simulink library "BLE_Library"  (R2017b)
settings: Solver=VariableStepAuto  StartTime=0.0  StopTime=10.0  RelTol=1e-3
values from neighbouring files (symbols this model uses):
  D = D/ScaleCoefficient    [BLE_PostLoad.m]    (also in new_BLE_model.m = zeros(N_BLE,N_BLE+1))
undefined symbols (not defined in the file or in its folder): ADV_IND_AccA, ADV_IND_id, BT_Hop_Separation, BT_Samples_Per_Symbol, CONNECT_IND_id, CONNECT_IND_length, F3B672D172DF, F506B10B1B3E, Header, LL_DATA_EMPTY_length, LL_DATA_id, magnitude, Payload, Preamble, Slot_Ts, T_IFS
libraries: BLE_Library x56, simulink x39, commutil2 x29, dspindex x17, commdigbbndfm2 x5, dspsigops x2, commrandsrc3 x2, dspstat3 x2, dspsrcs4 x1, dsparch4 x1, commdigbbndcpm2 x1
(part 3 of 5)

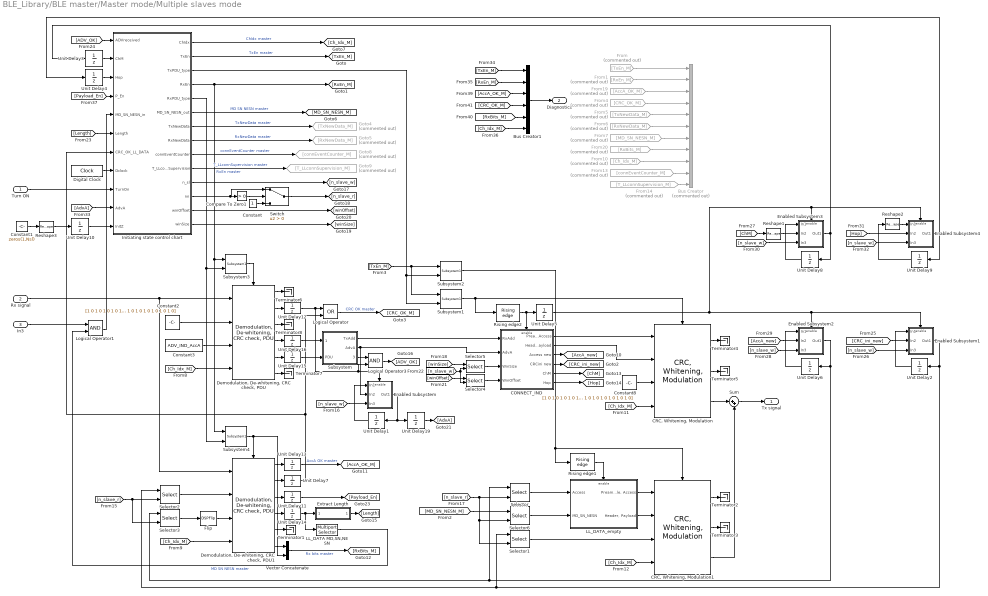
== system BLE_Library/BLE master/Master mode/Multiple slaves mode ==
  Turn ON : Inport
  Rx signal : Inport  Port=2
  In3 : Inport  Port=3
  Bus Creator : BusCreator  Commented=on  Inputs=11
  Bus Creator1 : BusCreator  Inputs=6
  CONNECT_IND : Subsystem
  "CRC, Whitening, Modulation" : BLE_Library/CRC, Whitening,  Modulation
  "CRC, Whitening, Modulation1" : BLE_Library/CRC, Whitening,  Modulation
  Compare To Zero1 : simulink/Logic and Bit Operations/Compare To Zero  relop=>  OutDataTypeStr=boolean
  Constant : Constant  SampleTime=-1
  Constant1 : Constant  Value=zeros(1,Nsl)  OutDataTypeStr=double  SampleTime=Slot_Ts
  Constant2 : Constant  Value=[1 0 1 0 1 0 1 0 1 0 1 0 1 0 1 0 1 0 1 0 1 0 1 0]  OutDataTypeStr=boolean  SampleTime=Slot_Ts
  Constant3 : Constant  Value=ADV_IND_AccA  VectorParams1D=off  SampleTime=Slot_Ts
  Constant8 : Constant  Value=[1 0 1 0 1 0 1 0 1 0 1 0 1 0 1 0 1 0 1 0 1 0 1 0]  OutDataTypeStr=boolean  SampleTime=Slot_Ts
  "Demodulation, De-whitening, CRC check, PDU" : BLE_Library/Demodulation, De-whitening, CRC check, PDU  PDU_Length=112 %ADV_DIRECT_IND: 2+6+6 octets (H,AdvA,TargetA)  N_after=136 %max PDU length + CRC
  "Demodulation, De-whitening, CRC check, PDU1" : BLE_Library/Demodulation, De-whitening, CRC check, PDU  PDU_Length=2 %PDU is not required  N_after=2080 %max PDU length + CRC: 16 + 255*8 + 24
  Digital Clock : DigitalClock  SampleTime=Slot_Ts
  Enabled Subsystem : Subsystem  TreatAsAtomicUnit=on
  Enabled Subsystem1 : Subsystem  TreatAsAtomicUnit=on
  Enabled Subsystem2 : Subsystem  TreatAsAtomicUnit=on
  Enabled Subsystem3 : Subsystem  TreatAsAtomicUnit=on
  Enabled Subsystem4 : Subsystem  TreatAsAtomicUnit=on
  Extract Length : Subsystem
      mask Display: disp('Extract length')
  Flip : DSPFlip
  From : From  Commented=on  GotoTag=TxEn_M
  From1 : From  Commented=on  GotoTag=RxEn_M
  From10 : From  Commented=on  GotoTag=Ch_Idx_M
  From13 : From  Commented=on  GotoTag=connEventCounter_M
  From14 : From  Commented=on  GotoTag=T_LLconnSupervision_M
  From19 : From  Commented=on  GotoTag=AccA_OK_M
  From20 : From  Commented=on  GotoTag=RxBits_M
  From4 : From  Commented=on  GotoTag=CRC_OK_M
  From5 : From  Commented=on  GotoTag=TxNewData_M
  From6 : From  Commented=on  GotoTag=RxNewData_M
  From7 : From  Commented=on  GotoTag=MD_SN_NESN_M
  Goto4 : Goto  Commented=on  GotoTag=TxNewData_M
  Goto5 : Goto  Commented=on  GotoTag=RxNewData_M
  Goto8 : Goto  Commented=on  GotoTag=connEventCounter_M
  Goto9 : Goto  Commented=on  GotoTag=T_LLconnSupervision_M
  Initiating state control chart : Stateflow chart  TreatAsAtomicUnit=on
  LL_DATA MD,SN,NESN : dspindex/Multiport Selector  rowsOrCols=Rows  idxCellArray={12:14}  idxErrMode=Clip Index
  LL_DATA_empty : Subsystem
  Logical Operator : Logic  Operator=OR  AllPortsSameDT=off  OutDataTypeStr=boolean
  Logical Operator1 : Logic  AllPortsSameDT=off  OutDataTypeStr=boolean
  Logical Operator3 : Logic  AllPortsSameDT=off  OutDataTypeStr=boolean
  Reshape1 : Reshape  OutputDimensionality=Column vector (2-D)
  Reshape2 : Reshape  OutputDimensionality=Row vector (2-D)
  Reshape3 : Reshape  OutputDimensionality=Row vector (2-D)
  Rising edge1 : BLE_Library/Rising edge  SystemSampleTime=-1
  Rising edge2 : BLE_Library/Rising edge  SystemSampleTime=-1
  Selector{,1..6} (7 alike) : Selector  NumberOfDimensions=2  InputPortWidth=3  IndexOptions=Select all,Index vector (port)  Indices=[1 3],2  OutputSizes=1,1
  Subsystem : Subsystem
  Subsystem1 : BLE_Library/Subsystem1  PDU_type=CONNECT_IND_id
  Subsystem2 : BLE_Library/Subsystem1  PDU_type=LL_DATA_id
  Subsystem3 : BLE_Library/Subsystem1  PDU_type=ADV_IND_id
  Subsystem4 : BLE_Library/Subsystem1  PDU_type=LL_DATA_id
  Sum : Sum  Inputs=|++
  Switch : Switch  Criteria=u2 > Threshold
  Terminator{1..8} (8 alike) : Terminator
  Unit Delay1 : UnitDelay  InitialCondition=zeros(48,Nsl)  SampleTime=Slot_Ts
  Unit Delay{3..5,7,10..16,19} (12 alike) : UnitDelay  SampleTime=Slot_Ts
  Unit Delay2 : UnitDelay  InitialCondition=zeros(24,Nsl)  SampleTime=Slot_Ts
  Unit Delay6 : UnitDelay  InitialCondition=zeros(32,Nsl)  SampleTime=Slot_Ts
  Unit Delay8 : UnitDelay  InitialCondition=zeros(40,Nsl)  SampleTime=Slot_Ts
  Unit Delay9 : UnitDelay  InitialCondition=zeros(1,Nsl)  SampleTime=Slot_Ts
  Vector Concatenate : Concatenate
  Tx signal : Outport
  Diagnostics : Outport  Port=2
  wires:
  "Demodulation, De-whitening, CRC check, PDU1"/2 -> Unit Delay7/1
  Subsystem4/1 -> "Demodulation, De-whitening, CRC check, PDU1"/Enable, Vector Concatenate/2
  Selector4/1 -> CONNECT_IND/4(WinOffset)
  [n_slave_w] -> Enabled Subsystem/3(In3)
  "CRC, Whitening, Modulation1"/2 -> Terminator3/1
  [Ch_Idx_M] -> "CRC, Whitening, Modulation1"/4
  Initiating state control chart/8(RxNewData) -> Goto5/1  "RxNewData master"
  Initiating state control chart/11(n_sl) -> [n_slave_w]
  "Demodulation, De-whitening, CRC check, PDU"/2 -> Unit Delay12/1
  Unit Delay12/1 -> Enabled Subsystem/Enable, Logical Operator3/2, Logical Operator/1
  Initiating state control chart/10(T_LLconnSupervision) -> Goto9/1  "T_LLconnSupervision master"
  Unit Delay19/1 -> [AdvA]
  [n_slave_w] -> Enabled Subsystem2/3(In3)
  Selector/1 -> LL_DATA_empty/1(Access)
  From/1 -> Bus Creator/1
  Subsystem/2(AdvA) -> CONNECT_IND/2(AdvA), Enabled Subsystem/2(In2)
  "Demodulation, De-whitening, CRC check, PDU"/1 -> Terminator6/1
  Initiating state control chart/9(connEventCounter) -> Goto8/1  "connEventCounter master"
  Sum/1 -> Tx signal/1
  CONNECT_IND/6(Hop) -> [Hop]
  [TxEn_M] -> Bus Creator1/1
  Enabled Subsystem/1(Out1) -> Unit Delay1/1, Unit Delay19/1
  Rising edge1/1 -> LL_DATA_empty/Enable
  Initiating state control chart/1(ChIdx) -> [Ch_Idx_M]  "ChIdx master"
  [RxBits_M] -> Bus Creator1/5
  Initiating state control chart/3(TxPDU_type) -> Subsystem2/2, Subsystem1/2
  LL_DATA_empty/1("Preamble, Access") -> "CRC, Whitening, Modulation1"/1
  Initiating state control chart/4(RxEn) -> [RxEn_M], Subsystem4/1, Subsystem3/1  "RxEn master"
  Subsystem/1(TxAdd) -> CONNECT_IND/1(RxAdd)
  Initiating state control chart/5(RxPDU_type) -> Subsystem4/2, Subsystem3/2
  From13/1 -> Bus Creator/10
  Initiating state control chart/6(MD_SN_NESN_out) -> [MD_SN_NESN_M]  "MD SN NESN master"
  [winOffset] -> Selector4/1
  From14/1 -> Bus Creator/11
  From4/1 -> Bus Creator/4
  Initiating state control chart/14(winSize) -> [winSize]
  [AccA_new] -> Enabled Subsystem2/2(In2)
  From20/1 -> Bus Creator/8
  Unit Delay6/1 -> Enabled Subsystem2/1(In1)
  "Demodulation, De-whitening, CRC check, PDU1"/1 -> Unit Delay13/1
  [Hop] -> Enabled Subsystem4/2(In2)
  Constant8/1 -> "CRC, Whitening, Modulation"/3
  Constant1/1 -> Reshape3/1
  Enabled Subsystem1/1(Out1) -> Unit Delay2/1, Selector2/1, Selector1/1
  Unit Delay7/1 -> Logical Operator/2, Initiating state control chart/7(CRC_OK_LL_DATA)
  Digital Clock/1 -> Initiating state control chart/8(Dclock)
  CONNECT_IND/4(CRCini new) -> [CRC_ini_new]
  Selector6/1 -> LL_DATA_empty/2(MD_SN_NESN)
  Initiating state control chart/13(winOffset) -> [winOffset]
  Enabled Subsystem3/1(Out1) -> Unit Delay3/1, Unit Delay8/1
  [n_slave_w] -> Enabled Subsystem4/3(In3)
  Unit Delay5/1 -> Enabled Subsystem2/Enable, Enabled Subsystem1/Enable, Enabled Subsystem4/Enable, Enabled Subsystem3/Enable
  Unit Delay16/1 -> Subsystem/1(Header)
  Compare To Zero1/1 -> Switch/2
  Enabled Subsystem4/1(Out1) -> Unit Delay4/1, Unit Delay9/1
  Enabled Subsystem2/1(Out1) -> Selector/1, Selector3/1, Unit Delay6/1
  [AccA_OK_M] -> Bus Creator1/3
  CONNECT_IND/5(ChM) -> [ChM]
  CONNECT_IND/3(Access new) -> [AccA_new]
  [MD_SN_NESN_M] -> Selector6/1
  Reshape2/1 -> Enabled Subsystem4/1(In1)
  "Demodulation, De-whitening, CRC check, PDU"/3 -> Terminator8/1
  Logical Operator/1 -> [CRC_OK_M]  "CRC OK master"
  Constant3/1 -> "Demodulation, De-whitening, CRC check, PDU"/3
  [Ch_Idx_M] -> "Demodulation, De-whitening, CRC check, PDU"/4
  Unit Delay9/1 -> Reshape2/1
  Switch/1 -> [n_slave_r]
  Unit Delay13/1 -> [AccA_OK_M]  "AccA OK master"
  From19/1 -> Bus Creator/3
  Turn ON/1 -> Initiating state control chart/9(TurnOn)
  [RxEn_M] -> Bus Creator1/2
  Subsystem/3(ADV OK) -> Logical Operator3/1
  Rx signal/1 -> "Demodulation, De-whitening, CRC check, PDU1"/1, "Demodulation, De-whitening, CRC check, PDU"/1
  Unit Delay1/1 -> Enabled Subsystem/1(In1)
  LL_DATA_empty/2("Header, Payload") -> "CRC, Whitening, Modulation1"/2
  Selector2/1 -> "Demodulation, De-whitening, CRC check, PDU1"/2
  From5/1 -> Bus Creator/5
  Unit Delay8/1 -> Enabled Subsystem3/1(In1)
  Initiating state control chart/7(TxNewData) -> Goto4/1  "TxNewData master"
  From1/1 -> Bus Creator/2
  Unit Delay10/1 -> Initiating state control chart/11(InitZ)
  [Ch_Idx_M] -> "CRC, Whitening, Modulation"/4
  Bus Creator1/1 -> Diagnostics/1
  From7/1 -> Bus Creator/7
  Unit Delay4/1 -> Initiating state control chart/3(Hop)
  [n_slave_w] -> Enabled Subsystem3/3(In3)
  Subsystem1/1 -> Rising edge2/1, "CRC, Whitening, Modulation"/Enable
  LL_DATA MD,SN,NESN/1 -> Logical Operator1/2  "MD SN NESN master"
  [n_slave_w] -> Enabled Subsystem1/3(In3)
  Reshape3/1 -> Unit Delay10/1
  Logical Operator3/1 -> [ADV_OK]
  "CRC, Whitening, Modulation"/3 -> Sum/1
  Selector3/1 -> Flip/1
  From6/1 -> Bus Creator/6
  "CRC, Whitening, Modulation1"/1 -> Terminator2/1
  [CRC_ini_new] -> Enabled Subsystem1/2(In2)
  Unit Delay2/1 -> Enabled Subsystem1/1(In1)
  Unit Delay14/1 -> Extract Length/1(Header), LL_DATA MD,SN,NESN/1
  "CRC, Whitening, Modulation1"/3 -> Sum/2
  Unit Delay15/1 -> Subsystem/2(PDU)
  Selector5/1 -> CONNECT_IND/3(WinSize)
  Reshape1/1 -> Enabled Subsystem3/2(In2)
  Constant2/1 -> "Demodulation, De-whitening, CRC check, PDU"/2
  [Payload_En] -> Initiating state control chart/4(P_En)
  "CRC, Whitening, Modulation"/2 -> Terminator5/1
  [n_slave_w] -> Selector4/2, Selector5/2
  [Ch_Idx_M] -> "Demodulation, De-whitening, CRC check, PDU1"/4
  Unit Delay3/1 -> Initiating state control chart/2(ChM)
  Initiating state control chart/2(TxEn) -> [TxEn_M]  "TxEn master"
  Vector Concatenate/1 -> [RxBits_M]  "Rx bits master"
  From10/1 -> Bus Creator/9
  Flip/1 -> "Demodulation, De-whitening, CRC check, PDU1"/3
  [AdvA] -> Initiating state control chart/10(AdvA)
  Selector1/1 -> "CRC, Whitening, Modulation1"/3
  Constant/1 -> Switch/3
  [ADV_OK] -> Initiating state control chart/1(ADVreceived)
  Subsystem2/1 -> Rising edge1/1, "CRC, Whitening, Modulation1"/Enable
  "Demodulation, De-whitening, CRC check, PDU"/6 -> Terminator7/1
  "Demodulation, De-whitening, CRC check, PDU1"/6 -> Vector Concatenate/1
  [ChM] -> Reshape1/1
  Subsystem3/1 -> "Demodulation, De-whitening, CRC check, PDU"/Enable
  Extract Length/1(Length) -> [Length]
  "Demodulation, De-whitening, CRC check, PDU"/5 -> Unit Delay15/1
  [winSize] -> Selector5/1
  [n_slave_r] -> Selector3/2, Selector2/2
  [TxEn_M] -> Subsystem2/1, Subsystem1/1
  [Length] -> Initiating state control chart/6(Length)
  CONNECT_IND/2("Header, Payload") -> "CRC, Whitening, Modulation"/2
  "Demodulation, De-whitening, CRC check, PDU1"/3 -> Unit Delay11/1
  "Demodulation, De-whitening, CRC check, PDU1"/5 -> Terminator1/1
  [Ch_Idx_M] -> Bus Creator1/6
  [CRC_OK_M] -> Bus Creator1/4
  "Demodulation, De-whitening, CRC check, PDU"/4 -> Unit Delay16/1
  Logical Operator1/1 -> Initiating state control chart/5(MD_SN_NESN_in)
  "CRC, Whitening, Modulation"/1 -> Terminator4/1
  "Demodulation, De-whitening, CRC check, PDU1"/4 -> Unit Delay14/1
  CONNECT_IND/1("Preamble, Access") -> "CRC, Whitening, Modulation"/1
  Initiating state control chart/12(nn) -> Compare To Zero1/1, Switch/1
  [n_slave_r] -> Selector/2, Selector1/2, Selector6/2
  Rising edge2/1 -> CONNECT_IND/Enable, Unit Delay5/1
  Unit Delay11/1 -> [Payload_En]
  In3/1 -> Logical Operator1/1

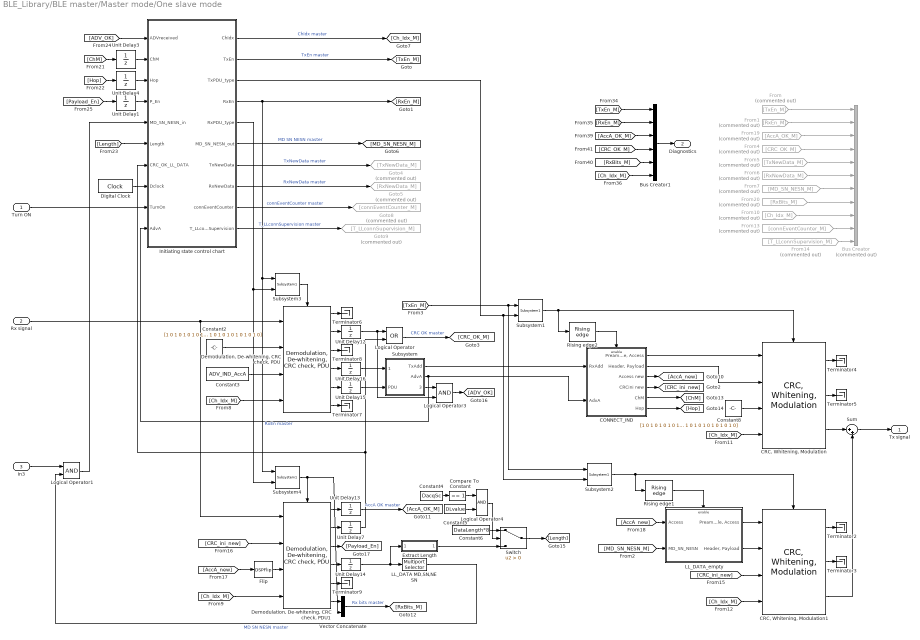
== system BLE_Library/BLE master/Master mode/One slave mode ==
  Turn ON : Inport
  Rx signal : Inport  Port=2
  In3 : Inport  Port=3
  Bus Creator : BusCreator  Commented=on  Inputs=11
  Bus Creator1 : BusCreator  Inputs=6
  CONNECT_IND : Subsystem
  "CRC, Whitening, Modulation" : BLE_Library/CRC, Whitening,  Modulation
  "CRC, Whitening, Modulation1" : BLE_Library/CRC, Whitening,  Modulation
  Compare To Constant : simulink/Logic and Bit Operations/Compare To Constant  relop===  const=1  OutDataTypeStr=boolean
  Constant2 : Constant  Value=[1 0 1 0 1 0 1 0 1 0 1 0 1 0 1 0 1 0 1 0 1 0 1 0]  OutDataTypeStr=boolean  SampleTime=Slot_Ts
  Constant3 : Constant  Value=ADV_IND_AccA  VectorParams1D=off  SampleTime=Slot_Ts
  Constant4 : Constant  Value=DacqSc  SampleTime=Slot_Ts
  Constant5 : Constant  Value=DLvalue  SampleTime=Slot_Ts
  Constant6 : Constant  Value=DataLength*8  SampleTime=Slot_Ts
  Constant8 : Constant  Value=[1 0 1 0 1 0 1 0 1 0 1 0 1 0 1 0 1 0 1 0 1 0 1 0]  OutDataTypeStr=boolean  SampleTime=Slot_Ts
  "Demodulation, De-whitening, CRC check, PDU" : BLE_Library/Demodulation, De-whitening, CRC check, PDU  PDU_Length=112 %ADV_DIRECT_IND: 2+6+6 octets (H,AdvA,TargetA)  N_after=136 %max PDU length + CRC
  "Demodulation, De-whitening, CRC check, PDU1" : BLE_Library/Demodulation, De-whitening, CRC check, PDU  PDU_Length=2 %PDU is not required  N_after=2080 %max PDU length + CRC: 16 + 255*8 + 24
  Digital Clock : DigitalClock  SampleTime=Slot_Ts
  Extract Length : Subsystem
      mask Display: disp('Extract length')
  Flip : DSPFlip
  From : From  Commented=on  GotoTag=TxEn_M
  From1 : From  Commented=on  GotoTag=RxEn_M
  From10 : From  Commented=on  GotoTag=Ch_Idx_M
  From13 : From  Commented=on  GotoTag=connEventCounter_M
  From14 : From  Commented=on  GotoTag=T_LLconnSupervision_M
  From19 : From  Commented=on  GotoTag=AccA_OK_M
  From20 : From  Commented=on  GotoTag=RxBits_M
  From4 : From  Commented=on  GotoTag=CRC_OK_M
  From5 : From  Commented=on  GotoTag=TxNewData_M
  From6 : From  Commented=on  GotoTag=RxNewData_M
  From7 : From  Commented=on  GotoTag=MD_SN_NESN_M
  Goto4 : Goto  Commented=on  GotoTag=TxNewData_M
  Goto5 : Goto  Commented=on  GotoTag=RxNewData_M
  Goto8 : Goto  Commented=on  GotoTag=connEventCounter_M
  Goto9 : Goto  Commented=on  GotoTag=T_LLconnSupervision_M
  Initiating state control chart : Stateflow chart  TreatAsAtomicUnit=on
  LL_DATA MD,SN,NESN : dspindex/Multiport Selector  rowsOrCols=Rows  idxCellArray={12:14}  idxErrMode=Clip Index
  LL_DATA_empty : Subsystem
  Logical Operator : Logic  Operator=OR  AllPortsSameDT=off  OutDataTypeStr=boolean
  Logical Operator1 : Logic  AllPortsSameDT=off  OutDataTypeStr=boolean
  Logical Operator3 : Logic  AllPortsSameDT=off  OutDataTypeStr=boolean
  Logical Operator4 : Logic  AllPortsSameDT=off  OutDataTypeStr=boolean
  Rising edge1 : BLE_Library/Rising edge  SystemSampleTime=-1
  Rising edge2 : BLE_Library/Rising edge  SystemSampleTime=-1
  Subsystem : Subsystem
  Subsystem1 : BLE_Library/Subsystem1  PDU_type=CONNECT_IND_id
  Subsystem2 : BLE_Library/Subsystem1  PDU_type=LL_DATA_id
  Subsystem3 : BLE_Library/Subsystem1  PDU_type=ADV_IND_id
  Subsystem4 : BLE_Library/Subsystem1  PDU_type=LL_DATA_id
  Sum : Sum  Inputs=|++
  Switch : Switch  Criteria=u2 > Threshold
  Terminator{2..9} (8 alike) : Terminator
  Unit Delay{1,3..4,7,12..16} (9 alike) : UnitDelay  SampleTime=Slot_Ts
  Vector Concatenate : Concatenate
  Tx signal : Outport
  Diagnostics : Outport  Port=2
  wires:
  Subsystem/1(TxAdd) -> CONNECT_IND/1(RxAdd)
  From4/1 -> Bus Creator/4
  Unit Delay15/1 -> Subsystem/2(PDU)
  [TxEn_M] -> Subsystem1/1, Subsystem2/1
  From/1 -> Bus Creator/1
  CONNECT_IND/1("Preamble, Access") -> "CRC, Whitening, Modulation"/1
  From7/1 -> Bus Creator/7
  "CRC, Whitening, Modulation"/2 -> Terminator5/1
  Unit Delay4/1 -> Initiating state control chart/3(Hop)
  From5/1 -> Bus Creator/5
  Logical Operator3/1 -> [ADV_OK]
  Initiating state control chart/10(T_LLconnSupervision) -> Goto9/1  "T_LLconnSupervision master"
  Sum/1 -> Tx signal/1
  Digital Clock/1 -> Initiating state control chart/8(Dclock)
  CONNECT_IND/2("Header, Payload") -> "CRC, Whitening, Modulation"/2
  Compare To Constant/1 -> Logical Operator4/1
  Subsystem1/1 -> "CRC, Whitening, Modulation"/Enable, Rising edge2/1
  Unit Delay7/1 -> Logical Operator/2, Initiating state control chart/7(CRC_OK_LL_DATA)
  [Ch_Idx_M] -> Bus Creator1/6
  In3/1 -> Logical Operator1/1
  Extract Length/1(Length) -> Switch/3
  [Hop] -> Unit Delay4/1
  CONNECT_IND/5(ChM) -> [ChM]
  "CRC, Whitening, Modulation"/3 -> Sum/1
  [Length] -> Initiating state control chart/6(Length)
  [AccA_OK_M] -> Bus Creator1/3
  [RxEn_M] -> Bus Creator1/2
  Initiating state control chart/5(RxPDU_type) -> Subsystem3/2, Subsystem4/2
  "Demodulation, De-whitening, CRC check, PDU"/4 -> Unit Delay16/1
  [CRC_ini_new] -> "CRC, Whitening, Modulation1"/3
  [Ch_Idx_M] -> "CRC, Whitening, Modulation"/4
  Unit Delay16/1 -> Subsystem/1(Header)
  "Demodulation, De-whitening, CRC check, PDU1"/4 -> Unit Delay14/1
  [Ch_Idx_M] -> "Demodulation, De-whitening, CRC check, PDU"/4
  "CRC, Whitening, Modulation"/1 -> Terminator4/1
  "Demodulation, De-whitening, CRC check, PDU"/5 -> Unit Delay15/1
  From14/1 -> Bus Creator/11
  [AccA_new] -> Flip/1
  LL_DATA_empty/1("Preamble, Access") -> "CRC, Whitening, Modulation1"/1
  Initiating state control chart/3(TxPDU_type) -> Subsystem1/2, Subsystem2/2
  [RxBits_M] -> Bus Creator1/5
  Initiating state control chart/4(RxEn) -> [RxEn_M], Subsystem3/1, Subsystem4/1  "RxEn master"
  CONNECT_IND/3(Access new) -> [AccA_new]
  Unit Delay1/1 -> Initiating state control chart/4(P_En)
  Rx signal/1 -> "Demodulation, De-whitening, CRC check, PDU1"/1, "Demodulation, De-whitening, CRC check, PDU"/1
  [ChM] -> Unit Delay3/1
  Subsystem4/1 -> "Demodulation, De-whitening, CRC check, PDU1"/Enable, Vector Concatenate/2
  "CRC, Whitening, Modulation1"/1 -> Terminator2/1
  LL_DATA_empty/2("Header, Payload") -> "CRC, Whitening, Modulation1"/2
  "Demodulation, De-whitening, CRC check, PDU"/6 -> Terminator7/1
  From13/1 -> Bus Creator/10
  [Ch_Idx_M] -> "CRC, Whitening, Modulation1"/4
  Constant5/1 -> Logical Operator4/2
  Bus Creator1/1 -> Diagnostics/1
  Vector Concatenate/1 -> [RxBits_M]  "Rx bits master"
  Unit Delay14/1 -> LL_DATA MD,SN,NESN/1, Extract Length/1(Header)
  "Demodulation, De-whitening, CRC check, PDU"/2 -> Unit Delay12/1
  "Demodulation, De-whitening, CRC check, PDU1"/3 -> [Payload_En]
  [AccA_new] -> LL_DATA_empty/1(Access)
  "CRC, Whitening, Modulation1"/2 -> Terminator3/1
  Initiating state control chart/1(ChIdx) -> [Ch_Idx_M]  "ChIdx master"
  "Demodulation, De-whitening, CRC check, PDU1"/1 -> Unit Delay13/1
  "Demodulation, De-whitening, CRC check, PDU"/3 -> Terminator8/1
  From19/1 -> Bus Creator/3
  Constant6/1 -> Switch/1
  [CRC_OK_M] -> Bus Creator1/4
  Unit Delay12/1 -> Logical Operator3/2, Logical Operator/1
  "Demodulation, De-whitening, CRC check, PDU1"/6 -> Vector Concatenate/1
  Initiating state control chart/9(connEventCounter) -> Goto8/1  "connEventCounter master"
  From1/1 -> Bus Creator/2
  Logical Operator1/1 -> Initiating state control chart/5(MD_SN_NESN_in)
  Subsystem3/1 -> "Demodulation, De-whitening, CRC check, PDU"/Enable
  [CRC_ini_new] -> "Demodulation, De-whitening, CRC check, PDU1"/2
  [Ch_Idx_M] -> "Demodulation, De-whitening, CRC check, PDU1"/4
  Constant2/1 -> "Demodulation, De-whitening, CRC check, PDU"/2
  Turn ON/1 -> Initiating state control chart/9(TurnOn)
  LL_DATA MD,SN,NESN/1 -> Logical Operator1/2  "MD SN NESN master"
  Rising edge1/1 -> LL_DATA_empty/Enable
  Initiating state control chart/8(RxNewData) -> Goto5/1  "RxNewData master"
  [TxEn_M] -> Bus Creator1/1
  Unit Delay13/1 -> [AccA_OK_M]  "AccA OK master"
  Initiating state control chart/2(TxEn) -> [TxEn_M]  "TxEn master"
  [Payload_En] -> Unit Delay1/1
  "Demodulation, De-whitening, CRC check, PDU1"/2 -> Unit Delay7/1
  From10/1 -> Bus Creator/9
  Unit Delay3/1 -> Initiating state control chart/2(ChM)
  [MD_SN_NESN_M] -> LL_DATA_empty/2(MD_SN_NESN)
  Logical Operator/1 -> [CRC_OK_M]  "CRC OK master"
  Initiating state control chart/6(MD_SN_NESN_out) -> [MD_SN_NESN_M]  "MD SN NESN master"
  Constant4/1 -> Compare To Constant/1
  "Demodulation, De-whitening, CRC check, PDU"/1 -> Terminator6/1
  CONNECT_IND/4(CRCini new) -> [CRC_ini_new]
  Subsystem2/1 -> Rising edge1/1, "CRC, Whitening, Modulation1"/Enable
  "Demodulation, De-whitening, CRC check, PDU1"/5 -> Terminator9/1
  [ADV_OK] -> Initiating state control chart/1(ADVreceived)
  Initiating state control chart/7(TxNewData) -> Goto4/1  "TxNewData master"
  From6/1 -> Bus Creator/6
  CONNECT_IND/6(Hop) -> [Hop]
  Switch/1 -> [Length]
  Constant3/1 -> "Demodulation, De-whitening, CRC check, PDU"/3
  Subsystem/3(ADV OK) -> Logical Operator3/1
  "CRC, Whitening, Modulation1"/3 -> Sum/2
  Flip/1 -> "Demodulation, De-whitening, CRC check, PDU1"/3
  Constant8/1 -> "CRC, Whitening, Modulation"/3
  Rising edge2/1 -> CONNECT_IND/Enable
  Logical Operator4/1 -> Switch/2
  Subsystem/2(AdvA) -> Initiating state control chart/10(AdvA), CONNECT_IND/2(AdvA)
  From20/1 -> Bus Creator/8

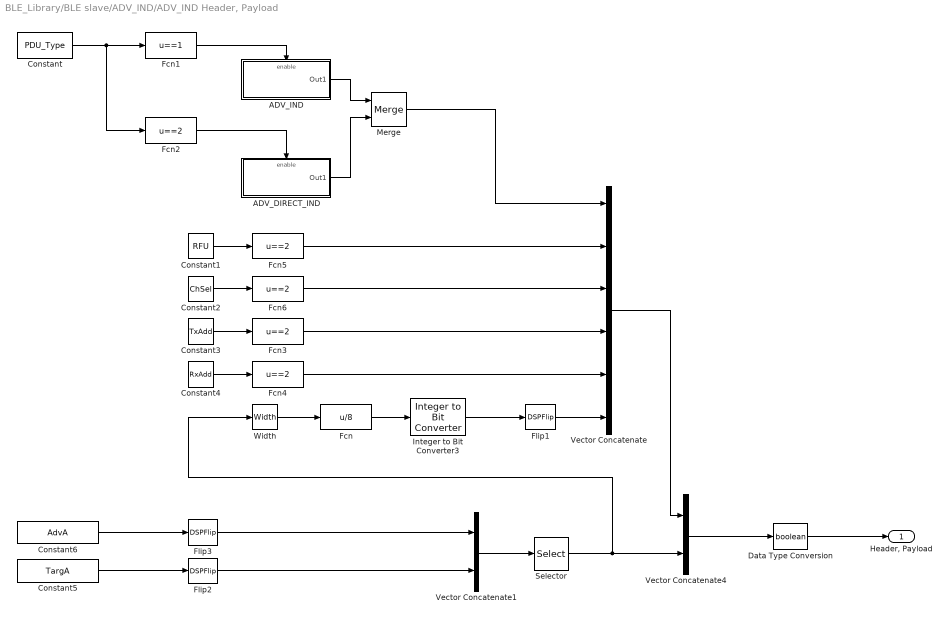
== system BLE_Library/BLE slave/ADV_IND/ADV_IND Header, Payload ==
  ADV_DIRECT_IND : Subsystem  TreatAsAtomicUnit=on
  ADV_IND : Subsystem  TreatAsAtomicUnit=on
  Constant : Constant  Value=PDU_Type  SampleTime=Slot_Ts
  Constant1 : Constant  Value=RFU  SampleTime=Slot_Ts
  Constant2 : Constant  Value=ChSel  SampleTime=Slot_Ts
  Constant3 : Constant  Value=TxAdd  SampleTime=Slot_Ts
  Constant4 : Constant  Value=RxAdd  SampleTime=Slot_Ts
  Constant5 : Constant  Value=TargA  VectorParams1D=off  OutDataTypeStr=double  SampleTime=Slot_Ts
  Constant6 : Constant  Value=AdvA  VectorParams1D=off  OutDataTypeStr=double  SampleTime=Slot_Ts
  Data Type Conversion : DataTypeConversion  OutDataTypeStr=boolean
  Fcn : Fcn  Expr=u/8
  Fcn1 : Fcn  Expr=u==1
  Fcn{2..6} (5 alike) : Fcn  Expr=u==2
  Flip1 : DSPFlip
  Flip2 : DSPFlip
  Flip3 : DSPFlip
  Integer to Bit Converter3 : commutil2/Integer to Bit Converter  nbits=8  signedInputValues=Unsigned  bitOrder=MSB first  outDtype=Inherit via internal rule
  Merge : Merge
  Selector : Selector  NumberOfDimensions=2  InputPortWidth=3  IndexOptions=Index vector (dialog),Index vector (dialog)  Indices=[1:48+48*(PDU_Type-1)],1  OutputSizes=1,1
  Vector Concatenate : Concatenate  NumInputs=6
  Vector Concatenate1 : Concatenate
  Vector Concatenate4 : Concatenate
  Width : Width
  "Header, Payload" : Outport
  wires:
  Data Type Conversion/1 -> "Header, Payload"/1
  Vector Concatenate/1 -> Vector Concatenate4/1
  Vector Concatenate4/1 -> Data Type Conversion/1
  Fcn/1 -> Integer to Bit Converter3/1
  Width/1 -> Fcn/1
  Vector Concatenate1/1 -> Selector/1
  Flip3/1 -> Vector Concatenate1/1
  Constant6/1 -> Flip3/1
  Flip1/1 -> Vector Concatenate/6
  Fcn5/1 -> Vector Concatenate/2
  Fcn6/1 -> Vector Concatenate/3
  Constant2/1 -> Fcn6/1
  Constant1/1 -> Fcn5/1
  Fcn4/1 -> Vector Concatenate/5
  Fcn3/1 -> Vector Concatenate/4
  Integer to Bit Converter3/1 -> Flip1/1
  Constant4/1 -> Fcn4/1
  Constant3/1 -> Fcn3/1
  Merge/1 -> Vector Concatenate/1
  ADV_DIRECT_IND/1(Out1) -> Merge/2
  ADV_IND/1(Out1) -> Merge/1
  Fcn2/1 -> ADV_DIRECT_IND/Enable
  Fcn1/1 -> ADV_IND/Enable
  Constant/1 -> Fcn1/1, Fcn2/1
  Constant5/1 -> Flip2/1
  Flip2/1 -> Vector Concatenate1/2
  Selector/1 -> Width/1, Vector Concatenate4/2

== system BLE_Library/BLE slave/ADV_IND/Subsystem4 ==
  AdvAccAdr1 : Constant  Value=ADV_IND_AccA  VectorParams1D=off  SampleTime=Slot_Ts
  AdvPreamble : Constant  Value=[0 1 0 1 0 1 0 1]'  VectorParams1D=off  OutDataTypeStr=boolean  SampleTime=Slot_Ts  FramePeriod=Slot_Ts
  "Concatenate Adv Preamble, Access address" : Concatenate  Mode=Multidimensional array
  Flip1 : DSPFlip
  Out1 : Outport
  wires:
  Flip1/1 -> "Concatenate Adv Preamble, Access address"/2
  AdvPreamble/1 -> "Concatenate Adv Preamble, Access address"/1
  "Concatenate Adv Preamble, Access address"/1 -> Out1/1
  AdvAccAdr1/1 -> Flip1/1

== system BLE_Library/BLE slave/Battery Status/Subsystem7 ==
  In1 : Inport
  MATLAB Function : MATLAB Function  TreatAsAtomicUnit=on
  Subsystem6 : Subsystem
      mask Display: disp('')
  Power level : Outport
  Time (h) to charge : Outport  Port=2
  Time (h) to discharge : Outport  Port=3
  wires:
  MATLAB Function/1(y) -> Power level/1
  In1/1 -> Subsystem6/1(In), MATLAB Function/1(u)
  Subsystem6/1(Time to charge (h)) -> Time (h) to charge/1
  Subsystem6/2(Time to discharge (h)) -> Time (h) to discharge/1

== system BLE_Library/BLE slave/Subsystem5/If Action Subsystem ==
  AdvA : Inport
  Action Port : ActionPort
  Compare To Constant : simulink/Logic and Bit Operations/Compare To Constant  relop===  const=48  OutDataTypeStr=boolean
  Constant2 : Constant  Value=AdvA  VectorParams1D=off  OutDataTypeStr=double  SampleTime=Slot_Ts
  Relational Operator1 : RelationalOperator  Operator===  OutDataTypeStr=boolean  RndMeth=Simplest
  Sum of Elements1 : Sum  Inputs=+
  CON OK : Outport
  wires:
  Relational Operator1/1 -> Sum of Elements1/1
  Sum of Elements1/1 -> Compare To Constant/1
  Constant2/1 -> Relational Operator1/1
  AdvA/1 -> Relational Operator1/2
  Compare To Constant/1 -> CON OK/1

== system BLE_Library/BLE slave/Subsystem5/If Action Subsystem1 ==
  AdvA : Inport
  InitA : Inport  Port=2
  Action Port : ActionPort
  Compare To Constant : simulink/Logic and Bit Operations/Compare To Constant  relop===  const=48  OutDataTypeStr=boolean
  Compare To Constant1 : simulink/Logic and Bit Operations/Compare To Constant  relop===  const=48  OutDataTypeStr=boolean
  Constant1 : Constant  Value=TargA  VectorParams1D=off  OutDataTypeStr=double  SampleTime=Slot_Ts
  Constant2 : Constant  Value=AdvA  VectorParams1D=off  OutDataTypeStr=double  SampleTime=Slot_Ts
  Logical Operator : Logic  AllPortsSameDT=off  OutDataTypeStr=boolean
  Relational Operator1 : RelationalOperator  Operator===  OutDataTypeStr=boolean  RndMeth=Simplest
  Relational Operator2 : RelationalOperator  Operator===  OutDataTypeStr=boolean  RndMeth=Simplest
  Sum of Elements1 : Sum  Inputs=+
  Sum of Elements2 : Sum  Inputs=+
  CON OK : Outport
  wires:
  Logical Operator/1 -> CON OK/1
  Compare To Constant/1 -> Logical Operator/1
  Sum of Elements1/1 -> Compare To Constant/1
  Relational Operator1/1 -> Sum of Elements1/1
  Constant2/1 -> Relational Operator1/1
  AdvA/1 -> Relational Operator1/2
  Sum of Elements2/1 -> Compare To Constant1/1
  Relational Operator2/1 -> Sum of Elements2/1
  InitA/1 -> Relational Operator2/1
  Constant1/1 -> Relational Operator2/2
  Compare To Constant1/1 -> Logical Operator/2

== system BLE_Library/CRC, Whitening, Modulation/Whitening/Initial LFSR ==
  ChIdx : Inport
  Enable : EnablePort  StatesWhenEnabling=reset
  Initial LFSR generation : MATLAB Function  TreatAsAtomicUnit=on
  LFSR : Outport
  wires:
  Initial LFSR generation/1(LFSR) -> LFSR/1
  ChIdx/1 -> Initial LFSR generation/1(ChIdx)

== system BLE_Library/Demodulation, De-whitening, CRC check, PDU/Access Code check, Payload read enable/AccA check ==
  Rx bits : Inport
  AccA : Inport  Port=2
  DataEn : EnablePort  StatesWhenEnabling=reset
  All 32 bits good : RelationalOperator  Operator===  RndMeth=Nearest  InputSameDT=on
  Constant : Constant  Value=32  SampleTime=Slot_Ts
  Relational Operator : RelationalOperator  Operator===  RndMeth=Nearest  InputSameDT=on
  Tapped Delay : simulink/Discrete/Tapped Delay  vinit=0.0  samptime=Slot_Ts  NumDelays=31  DelayOrder=Newest  includeCurrent=on
  Total correct bits : Sum  Inputs=1  OutDataTypeStr=double  SaturateOnIntegerOverflow=on  InputSameDT=on
  AccA OK : Outport  OutputWhenDisabled=reset  InitialOutput=0
  wires:
  AccA/1 -> Relational Operator/2
  Constant/1 -> All 32 bits good/2
  All 32 bits good/1 -> AccA OK/1
  Relational Operator/1 -> Total correct bits/1
  Total correct bits/1 -> All 32 bits good/1
  Rx bits/1 -> Tapped Delay/1
  Tapped Delay/1 -> Relational Operator/1

== system BLE_Library/Demodulation, De-whitening, CRC check, PDU/De-whitening, CRC check, Data fields/CRC calculation1 ==
  Payload : Inport
  CRC_ini : Inport  Port=2
  Enable : EnablePort  StatesWhenEnabling=reset
  CRC generation : MATLAB Function  TreatAsAtomicUnit=on
  Constant3 : Constant  SampleTime=Slot_Ts
  Flip : DSPFlip
  Switch : Switch  Criteria=u2 > Threshold
  Unit Delay1 : UnitDelay  SampleTime=Slot_Ts
  Unit Delay8 : UnitDelay  SampleTime=Slot_Ts
  CRC : Outport
  wires:
  Payload/1 -> CRC generation/1(bin)
  Unit Delay1/1 -> Switch/2
  Constant3/1 -> Unit Delay1/1
  CRC generation/1(CRC) -> Unit Delay8/1, Flip/1
  CRC_ini/1 -> Switch/3
  Unit Delay8/1 -> Switch/1
  Switch/1 -> CRC generation/2(LFSR)
  Flip/1 -> CRC/1

== system BLE_Library/Demodulation, De-whitening, CRC check, PDU/De-whitening, CRC check, Data fields/CRC comparison ==
  CRC calculated : Inport
  CRC received : Inport  Port=2
  Enable : EnablePort  StatesWhenEnabling=reset
  CRC comparison : Subsystem  TreatAsAtomicUnit=on
  Compare To Constant : simulink/Logic and Bit Operations/Compare To Constant  relop===  const=23  OutDataTypeStr=boolean
  Counter Free-Running : simulink/Sources/Counter Free-Running  NumBits=32  tsamp=Slot_Ts
  Tapped Delay1 : simulink/Discrete/Tapped Delay  vinit=0.0  samptime=Slot_Ts  NumDelays=23  DelayOrder=Oldest  includeCurrent=on
  CRC_OK : Outport  OutputWhenDisabled=reset  InitialOutput=0
  wires:
  CRC comparison/1(CRC_OK) -> CRC_OK/1
  CRC calculated/1 -> CRC comparison/1(CRC calculated)
  Compare To Constant/1 -> CRC comparison/Enable
  Tapped Delay1/1 -> CRC comparison/2(CRC received)
  CRC received/1 -> Tapped Delay1/1
  Counter Free-Running/1 -> Compare To Constant/1

== system BLE_Library/Demodulation, De-whitening, CRC check, PDU/De-whitening, CRC check, Data fields/Data ==
  In1 : Inport
  Enable : EnablePort  StatesWhenEnabling=reset
  PDU : Outport
  wires:
  In1/1 -> PDU/1

== system BLE_Library/Demodulation, De-whitening, CRC check, PDU/De-whitening, CRC check, Data fields/De-whitening ==
  Payload W : Inport
  ChIdx : Inport  Port=2
  Constant3 : Constant  SampleTime=Slot_Ts
  De-whitening : MATLAB Function  TreatAsAtomicUnit=on
  Subsystem : Subsystem
  Switch : Switch  Criteria=u2 > Threshold
  Unit Delay1 : UnitDelay  SampleTime=Slot_Ts
  Unit Delay8 : UnitDelay  SampleTime=Slot_Ts
  Payload : Outport
  wires:
  De-whitening/1(bout) -> Payload/1
  Unit Delay8/1 -> Switch/1
  De-whitening/2(LFSR_new) -> Unit Delay8/1
  Payload W/1 -> De-whitening/1(bin)
  Unit Delay1/1 -> Switch/2
  Switch/1 -> De-whitening/2(LFSR)
  Constant3/1 -> Unit Delay1/1, Subsystem/Enable
  ChIdx/1 -> Subsystem/1(ChIdx)
  Subsystem/1(LFSR) -> Switch/3

== system BLE_Library/Demodulation, De-whitening, CRC check, PDU/De-whitening, CRC check, Data fields/Get length ==
  In1 : Inport
  Enable : EnablePort  StatesWhenEnabling=reset
  Bit to Integer Converter : commutil2/Bit to Integer Converter  nbits=8  bitOrder=MSB first  signedOutputValues=Unsigned  outDtype=Inherit via internal rule  outDtypeSigned=Inherit via internal rule
  Constant : Constant  Value=8  SampleTime=Slot_Ts
  Multiport Selector : dspindex/Multiport Selector  rowsOrCols=Rows  idxCellArray={1:8}  idxErrMode=Clip Index
  Product : Product
  L : Outport
  H : Outport  Port=2
  wires:
  Constant/1 -> Product/1
  Bit to Integer Converter/1 -> Product/2
  Product/1 -> L/1
  Multiport Selector/1 -> Bit to Integer Converter/1
  In1/1 -> H/1, Multiport Selector/1

== system BLE_Library/Demodulation, De-whitening, CRC check, PDU/De-whitening, CRC check, Data fields/Store header ==
  P : Inport
  Enable : EnablePort  StatesWhenEnabling=reset
  Tapped Delay1 : simulink/Discrete/Tapped Delay  vinit=0.0  samptime=Slot_Ts  NumDelays=15  DelayOrder=Newest  includeCurrent=on
  H : Outport
  wires:
  P/1 -> Tapped Delay1/1
  Tapped Delay1/1 -> H/1

== system BLE_Library/Diagnostics/Bit Error Rate/Enabled Subsystem1 ==
  In1 : Inport
  Enable : EnablePort
  Out1 : Outport
  wires:
  In1/1 -> Out1/1

== system BLE_Library/Diagnostics/Packet Error Rate/Enabled Subsystem ==
  In1 : Inport
  Enable : EnablePort
  Out1 : Outport
  wires:
  In1/1 -> Out1/1

== system BLE_Library/Diagnostics/Packet Rejection Rate/Enabled Subsystem1 ==
  In1 : Inport
  Enable : EnablePort
  Out1 : Outport
  wires:
  In1/1 -> Out1/1

== system BLE_Library/802.11b interferer/Poisson pulses/If Action Subsystem1/Enabled Subsystem ==
  In1 : Inport
  In2 : Inport  Port=2
  Enable : EnablePort  StatesWhenEnabling=reset
  Out1 : Outport  InitialOutput=0
  Out2 : Outport  Port=2  InitialOutput=0
  wires:
  In1/1 -> Out1/1
  In2/1 -> Out2/1

== system BLE_Library/802.11b interferer/Poisson pulses/If Action Subsystem1/Enabled Subsystem1 ==
  In1 : Inport
  In2 : Inport  Port=2
  Enable : EnablePort
  Sum : Sum  Inputs=|++
  Out1 : Outport  InitialOutput=0
  wires:
  In1/1 -> Sum/1
  In2/1 -> Sum/2
  Sum/1 -> Out1/1

== system BLE_Library/802.11b interferer/Poisson pulses/If Action Subsystem1/Enabled Subsystem2 ==
  Enable : EnablePort  StatesWhenEnabling=reset
  Constant1 : Constant  Value=(packet_length)/Slot_Ts+1  SampleTime=Slot_Ts
  Constant2 : Constant  SampleTime=Slot_Ts
  Relational Operator : RelationalOperator  Operator=<  OutDataTypeStr=boolean  RndMeth=Simplest
  Sum : Sum  Inputs=|++
  Unit Delay1 : UnitDelay  InitialCondition=1  SampleTime=Slot_Ts
  Out3 : Outport  InitialOutput=0
  wires:
  Constant2/1 -> Sum/1
  Unit Delay1/1 -> Sum/2
  Sum/1 -> Relational Operator/1, Unit Delay1/1
  Constant1/1 -> Relational Operator/2
  Relational Operator/1 -> Out3/1

== system BLE_Library/BLE master/Master mode/Multiple slaves mode/CONNECT_IND ==
  RxAdd : Inport
  AdvA : Inport  Port=2
  WinSize : Inport  Port=3
  WinOffset : Inport  Port=4
  Enable : EnablePort  StatesWhenEnabling=reset
  "CONNECT_IND Header, Payload" : Subsystem
  Subsystem4 : Subsystem
      mask Display: disp('Adv\nPreamble,\nAccess')
  "Preamble, Access" : Outport  InitialOutput=0
  "Header, Payload" : Outport  Port=2  InitialOutput=0
  Access new : Outport  Port=3  InitialOutput=0
  CRCini new : Outport  Port=4  InitialOutput=0
  ChM : Outport  Port=5  InitialOutput=0
  Hop : Outport  Port=6  InitialOutput=0
  wires:
  WinOffset/1 -> "CONNECT_IND Header, Payload"/4(WinOffset)
  WinSize/1 -> "CONNECT_IND Header, Payload"/3(WinSize)
  "CONNECT_IND Header, Payload"/5(Hop) -> Hop/1
  "CONNECT_IND Header, Payload"/4(ChM) -> ChM/1
  "CONNECT_IND Header, Payload"/3(CRCini new) -> CRCini new/1
  "CONNECT_IND Header, Payload"/2(Access new) -> Access new/1
  RxAdd/1 -> "CONNECT_IND Header, Payload"/2(RxAdd)
  "CONNECT_IND Header, Payload"/1("Header, Payload") -> "Header, Payload"/1
  Subsystem4/1(Out1) -> "Preamble, Access"/1
  AdvA/1 -> "CONNECT_IND Header, Payload"/1(AdvA)

== system BLE_Library/BLE master/Master mode/Multiple slaves mode/Enabled Subsystem ==
  In1 : Inport
  In2 : Inport  Port=2
  In3 : Inport  Port=3
  Enable : EnablePort
  Assignment : Assignment  NumberOfDimensions=2  DiagnosticForDimensions=Warning  IndexOptions=Assign all,Index vector (port)  Indices=1,1  OutputSizes=1,1
  Out1 : Outport
  wires:
  Assignment/1 -> Out1/1
  In3/1 -> Assignment/3
  In2/1 -> Assignment/2
  In1/1 -> Assignment/1

== system BLE_Library/BLE master/Master mode/Multiple slaves mode/Enabled Subsystem1 ==
  In1 : Inport
  In2 : Inport  Port=2
  In3 : Inport  Port=3
  Enable : EnablePort
  Assignment : Assignment  NumberOfDimensions=2  DiagnosticForDimensions=Warning  IndexOptions=Assign all,Index vector (port)  Indices=1,1  OutputSizes=1,1
  Out1 : Outport
  wires:
  Assignment/1 -> Out1/1
  In3/1 -> Assignment/3
  In2/1 -> Assignment/2
  In1/1 -> Assignment/1

== system BLE_Library/BLE master/Master mode/Multiple slaves mode/Enabled Subsystem2 ==
  In1 : Inport
  In2 : Inport  Port=2
  In3 : Inport  Port=3
  Enable : EnablePort
  Assignment : Assignment  NumberOfDimensions=2  DiagnosticForDimensions=Warning  IndexOptions=Assign all,Index vector (port)  Indices=1,1  OutputSizes=1,1
  Out1 : Outport
  wires:
  Assignment/1 -> Out1/1
  In3/1 -> Assignment/3
  In2/1 -> Assignment/2
  In1/1 -> Assignment/1

== system BLE_Library/BLE master/Master mode/Multiple slaves mode/Enabled Subsystem3 ==
  In1 : Inport
  In2 : Inport  Port=2
  In3 : Inport  Port=3
  Enable : EnablePort
  Assignment : Assignment  NumberOfDimensions=2  DiagnosticForDimensions=Warning  IndexOptions=Assign all,Index vector (port)  Indices=1,1  OutputSizes=1,1
  Out1 : Outport
  wires:
  Assignment/1 -> Out1/1
  In3/1 -> Assignment/3
  In2/1 -> Assignment/2
  In1/1 -> Assignment/1

== system BLE_Library/BLE master/Master mode/Multiple slaves mode/Enabled Subsystem4 ==
  In1 : Inport
  In2 : Inport  Port=2
  In3 : Inport  Port=3
  Enable : EnablePort
  Assignment : Assignment  NumberOfDimensions=2  DiagnosticForDimensions=Warning  IndexOptions=Assign all,Index vector (port)  Indices=1,1  OutputSizes=1,1
  Out1 : Outport
  wires:
  Assignment/1 -> Out1/1
  In3/1 -> Assignment/3
  In2/1 -> Assignment/2
  In1/1 -> Assignment/1

== system BLE_Library/BLE master/Master mode/Multiple slaves mode/Extract Length ==
  Header : Inport
  Bit to Integer Converter : commutil2/Bit to Integer Converter  nbits=8  bitOrder=MSB first  signedOutputValues=Unsigned  outDtype=Inherit via internal rule  outDtypeSigned=Inherit via internal rule
  Constant : Constant  Value=8  SampleTime=Slot_Ts
  Multiport Selector : dspindex/Multiport Selector  rowsOrCols=Rows  idxCellArray={1:8}  idxErrMode=Clip Index
  Product : Product
  Length : Outport
  wires:
  Multiport Selector/1 -> Bit to Integer Converter/1
  Constant/1 -> Product/1
  Bit to Integer Converter/1 -> Product/2
  Header/1 -> Multiport Selector/1
  Product/1 -> Length/1

== system BLE_Library/BLE master/Master mode/Multiple slaves mode/LL_DATA_empty ==
  Access : Inport
  MD_SN_NESN : Inport  Port=2
  Enable : EnablePort  StatesWhenEnabling=reset
  "Concatenate Preamble, Access address" : Concatenate  Mode=Multidimensional array
  Flip : DSPFlip
  Header : Concatenate  NumInputs=4  Mode=Multidimensional array
  LLID : Constant  Value=[1 0]'  OutDataTypeStr=boolean  SampleTime=Slot_Ts
  Length : Constant  Value=[0 0 0 0 0 0 0 0]'  OutDataTypeStr=boolean  SampleTime=Slot_Ts
  MATLAB Function : MATLAB Function  TreatAsAtomicUnit=on
  RFU : Constant  Value=[0 0 0]'  OutDataTypeStr=boolean  SampleTime=Slot_Ts
  "Preamble, Access" : Outport  InitialOutput=0
  "Header, Payload" : Outport  Port=2  InitialOutput=0
  wires:
  Flip/1 -> Header/2
  RFU/1 -> Header/3
  Length/1 -> Header/4
  MD_SN_NESN/1 -> Flip/1
  Header/1 -> "Header, Payload"/1
  LLID/1 -> Header/1
  "Concatenate Preamble, Access address"/1 -> "Preamble, Access"/1
  MATLAB Function/1(Preamble) -> "Concatenate Preamble, Access address"/1
  Access/1 -> MATLAB Function/1(AccessAddress), "Concatenate Preamble, Access address"/2

== system BLE_Library/BLE master/Master mode/Multiple slaves mode/Subsystem ==
  Header : Inport
  PDU : Inport  Port=2
  ADV_IND : Constant  Value=[0 0 0 0]'  OutDataTypeStr=boolean  SampleTime=Slot_Ts
  If : If  IfExpression=u1 > 3
  If Action Subsystem : Subsystem  TreatAsAtomicUnit=on
  If Action Subsystem1 : Subsystem  TreatAsAtomicUnit=on
  Merge : Merge
  Merge1 : Merge
  Merge2 : Merge
  PDU Type : dspindex/Multiport Selector  rowsOrCols=Rows  idxCellArray={13:16}  idxErrMode=Clip Index
  Relational Operator : RelationalOperator  Operator===  OutDataTypeStr=boolean  RndMeth=Simplest
  Sum of Elements : Sum  Inputs=+
  TxAdd : Outport
  AdvA : Outport  Port=2
  ADV OK : Outport  Port=3
  wires:
  Merge2/1 -> ADV OK/1
  If Action Subsystem/3(ADV OK) -> Merge2/1
  If Action Subsystem1/1(ADV OK) -> Merge2/2
  If Action Subsystem/2(AdvA) -> Merge1/1
  PDU Type/1 -> Relational Operator/2
  ADV_IND/1 -> Relational Operator/1
  If Action Subsystem1/2(AdvA) -> Merge1/2
  If Action Subsystem1/3(TxAdd) -> Merge/2
  If/1 -> If Action Subsystem/Action
  Sum of Elements/1 -> If/1
  Relational Operator/1 -> Sum of Elements/1
  PDU/1 -> If Action Subsystem1/2(PDU), If Action Subsystem/2(PDU)
  If Action Subsystem/1(TxAdd) -> Merge/1
  Header/1 -> If Action Subsystem1/1(Header), If Action Subsystem/1(Header), PDU Type/1
  Merge1/1 -> AdvA/1
  Merge/1 -> TxAdd/1
  If/2 -> If Action Subsystem1/Action

== system BLE_Library/BLE master/Master mode/One slave mode/CONNECT_IND ==
  RxAdd : Inport
  AdvA : Inport  Port=2
  Enable : EnablePort  StatesWhenEnabling=reset
  "CONNECT_IND Header, Payload" : Subsystem
  Subsystem4 : Subsystem
      mask Display: disp('Adv\nPreamble,\nAccess')
  "Preamble, Access" : Outport  InitialOutput=0
  "Header, Payload" : Outport  Port=2  InitialOutput=0
  Access new : Outport  Port=3  InitialOutput=0
  CRCini new : Outport  Port=4  InitialOutput=0
  ChM : Outport  Port=5  InitialOutput=0
  Hop : Outport  Port=6  InitialOutput=0
  wires:
  "CONNECT_IND Header, Payload"/5(Hop) -> Hop/1
  "CONNECT_IND Header, Payload"/4(ChM) -> ChM/1
  "CONNECT_IND Header, Payload"/3(CRCini new) -> CRCini new/1
  "CONNECT_IND Header, Payload"/2(Access new) -> Access new/1
  RxAdd/1 -> "CONNECT_IND Header, Payload"/2(RxAdd)
  "CONNECT_IND Header, Payload"/1("Header, Payload") -> "Header, Payload"/1
  Subsystem4/1(Out1) -> "Preamble, Access"/1
  AdvA/1 -> "CONNECT_IND Header, Payload"/1(AdvA)

== system BLE_Library/BLE master/Master mode/One slave mode/Extract Length ==
  Header : Inport
  Bit to Integer Converter : commutil2/Bit to Integer Converter  nbits=8  bitOrder=MSB first  signedOutputValues=Unsigned  outDtype=Inherit via internal rule  outDtypeSigned=Inherit via internal rule
  Constant : Constant  Value=8  SampleTime=Slot_Ts
  Multiport Selector : dspindex/Multiport Selector  rowsOrCols=Rows  idxCellArray={1:8}  idxErrMode=Clip Index
  Product : Product
  Length : Outport
  wires:
  Multiport Selector/1 -> Bit to Integer Converter/1
  Constant/1 -> Product/1
  Bit to Integer Converter/1 -> Product/2
  Header/1 -> Multiport Selector/1
  Product/1 -> Length/1

== system BLE_Library/BLE master/Master mode/One slave mode/LL_DATA_empty ==
  Access : Inport
  MD_SN_NESN : Inport  Port=2
  Enable : EnablePort  StatesWhenEnabling=reset
  "Concatenate Preamble, Access address" : Concatenate  Mode=Multidimensional array
  Flip : DSPFlip
  Header : Concatenate  NumInputs=4  Mode=Multidimensional array
  LLID : Constant  Value=[1 0]'  OutDataTypeStr=boolean  SampleTime=Slot_Ts
  Length : Constant  Value=[0 0 0 0 0 0 0 0]'  OutDataTypeStr=boolean  SampleTime=Slot_Ts
  MATLAB Function : MATLAB Function  TreatAsAtomicUnit=on
  RFU : Constant  Value=[0 0 0]'  OutDataTypeStr=boolean  SampleTime=Slot_Ts
  "Preamble, Access" : Outport  InitialOutput=0
  "Header, Payload" : Outport  Port=2  InitialOutput=0
  wires:
  Flip/1 -> Header/2
  RFU/1 -> Header/3
  Length/1 -> Header/4
  MD_SN_NESN/1 -> Flip/1
  Header/1 -> "Header, Payload"/1
  LLID/1 -> Header/1
  "Concatenate Preamble, Access address"/1 -> "Preamble, Access"/1
  MATLAB Function/1(Preamble) -> "Concatenate Preamble, Access address"/1
  Access/1 -> MATLAB Function/1(AccessAddress), "Concatenate Preamble, Access address"/2

== system BLE_Library/BLE master/Master mode/One slave mode/Subsystem ==
  Header : Inport
  PDU : Inport  Port=2
  ADV_IND : Constant  Value=[0 0 0 0]'  OutDataTypeStr=boolean  SampleTime=Slot_Ts
  If : If  IfExpression=u1 > 3
  If Action Subsystem : Subsystem  TreatAsAtomicUnit=on
  If Action Subsystem1 : Subsystem  TreatAsAtomicUnit=on
  Merge : Merge
  Merge1 : Merge
  Merge2 : Merge
  PDU Type : dspindex/Multiport Selector  rowsOrCols=Rows  idxCellArray={13:16}  idxErrMode=Clip Index
  Relational Operator : RelationalOperator  Operator===  OutDataTypeStr=boolean  RndMeth=Simplest
  Sum of Elements : Sum  Inputs=+
  TxAdd : Outport
  AdvA : Outport  Port=2
  ADV OK : Outport  Port=3
  wires:
  Merge2/1 -> ADV OK/1
  If Action Subsystem/3(ADV OK) -> Merge2/1
  If Action Subsystem1/1(ADV OK) -> Merge2/2
  If Action Subsystem/2(AdvA) -> Merge1/1
  PDU Type/1 -> Relational Operator/2
  ADV_IND/1 -> Relational Operator/1
  If Action Subsystem1/2(AdvA) -> Merge1/2
  If Action Subsystem1/3(TxAdd) -> Merge/2
  If/1 -> If Action Subsystem/Action
  Sum of Elements/1 -> If/1
  Relational Operator/1 -> Sum of Elements/1
  PDU/1 -> If Action Subsystem1/2(PDU), If Action Subsystem/2(PDU)
  If Action Subsystem/1(TxAdd) -> Merge/1
  Header/1 -> If Action Subsystem1/1(Header), If Action Subsystem/1(Header), PDU Type/1
  Merge1/1 -> AdvA/1
  Merge/1 -> TxAdd/1
  If/2 -> If Action Subsystem1/Action

== system BLE_Library/BLE slave/ADV_IND/ADV_IND Header, Payload/ADV_DIRECT_IND ==
  Enable : EnablePort
  ADV_DIRECT_IND : Constant  Value=[1 0 0 0]'  VectorParams1D=off  SampleTime=Slot_Ts  FramePeriod=Slot_Ts
  Out1 : Outport
  wires:
  ADV_DIRECT_IND/1 -> Out1/1

== system BLE_Library/BLE slave/ADV_IND/ADV_IND Header, Payload/ADV_IND ==
  Enable : EnablePort
  ADV_IND : Constant  Value=[0 0 0 0]'  VectorParams1D=off  SampleTime=Slot_Ts  FramePeriod=Slot_Ts
  Out1 : Outport
  wires:
  ADV_IND/1 -> Out1/1

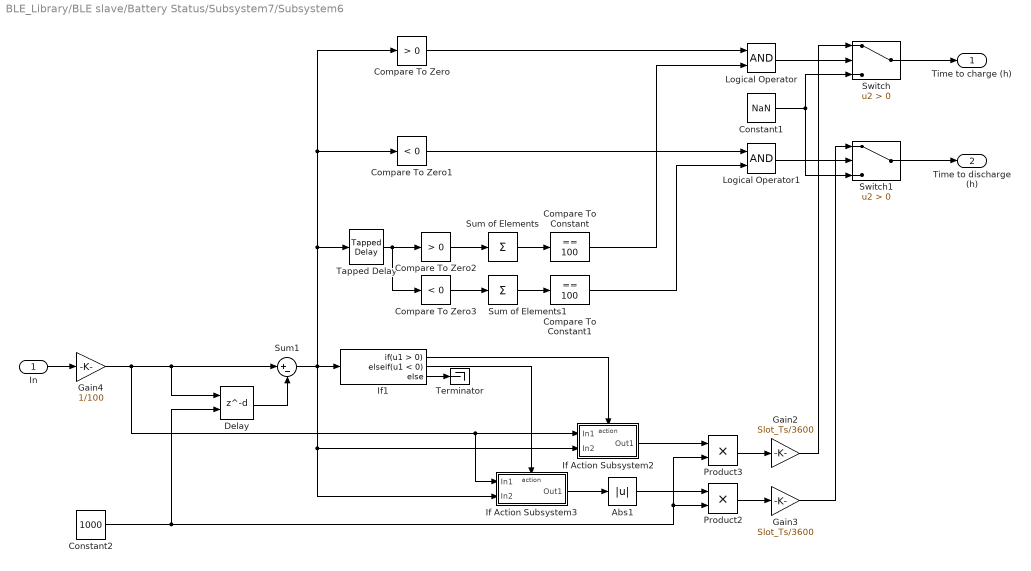
== system BLE_Library/BLE slave/Battery Status/Subsystem7/Subsystem6 ==
  In : Inport
  Abs1 : Abs
  Compare To Constant : simulink/Logic and Bit Operations/Compare To Constant  relop===  const=100  OutDataTypeStr=boolean
  Compare To Constant1 : simulink/Logic and Bit Operations/Compare To Constant  relop===  const=100  OutDataTypeStr=boolean
  Compare To Zero : simulink/Logic and Bit Operations/Compare To Zero  relop=>  OutDataTypeStr=boolean
  Compare To Zero1 : simulink/Logic and Bit Operations/Compare To Zero  relop=<  OutDataTypeStr=boolean
  Compare To Zero2 : simulink/Logic and Bit Operations/Compare To Zero  relop=>  OutDataTypeStr=boolean
  Compare To Zero3 : simulink/Logic and Bit Operations/Compare To Zero  relop=<  OutDataTypeStr=boolean
  Constant1 : Constant  Value=NaN  SampleTime=-1
  Constant2 : Constant  Value=1000  SampleTime=Slot_Ts
  Delay : Delay  DelayLengthSource=Input port  DelayLengthUpperLimit=10000  InitialCondition=1  SampleTime=Slot_Ts
      settings: InputPortMap=u0,p1
  Gain2 : Gain  Gain=Slot_Ts/3600
  Gain3 : Gain  Gain=Slot_Ts/3600
  Gain4 : Gain  Gain=1/100
  If Action Subsystem2 : Subsystem  TreatAsAtomicUnit=on
  If Action Subsystem3 : Subsystem  TreatAsAtomicUnit=on
  If1 : If  ElseIfExpressions=u1 < 0
  Logical Operator : Logic  AllPortsSameDT=off  OutDataTypeStr=boolean
  Logical Operator1 : Logic  AllPortsSameDT=off  OutDataTypeStr=boolean
  Product2 : Product
  Product3 : Product
  Sum of Elements : Sum  Inputs=+
  Sum of Elements1 : Sum  Inputs=+
  Sum1 : Sum  Inputs=|+-
  Switch : Switch  Criteria=u2 > Threshold
  Switch1 : Switch  Criteria=u2 > Threshold
  Tapped Delay : simulink/Discrete/Tapped Delay  vinit=0.0  samptime=Slot_Ts  NumDelays=99  DelayOrder=Oldest  includeCurrent=on
  Terminator : Terminator
  Time to charge (h) : Outport
  Time to discharge (h) : Outport  Port=2
  wires:
  In/1 -> Gain4/1
  Gain4/1 -> Delay/1, Sum1/1, If Action Subsystem3/1(In1), If Action Subsystem2/1(In1)
  Delay/1 -> Sum1/2
  Sum1/1 -> Tapped Delay/1, Compare To Zero/1, Compare To Zero1/1, If Action Subsystem3/2(In2), If Action Subsystem2/2(In2), If1/1
  If1/1 -> If Action Subsystem2/Action
  If1/2 -> If Action Subsystem3/Action
  If Action Subsystem3/1(Out1) -> Abs1/1
  Product3/1 -> Gain2/1
  Product2/1 -> Gain3/1
  If Action Subsystem2/1(Out1) -> Product3/1
  Abs1/1 -> Product2/1
  Constant2/1 -> Delay/2, Product3/2, Product2/2
  Gain2/1 -> Switch/1
  Constant1/1 -> Switch1/3, Switch/3
  Switch/1 -> Time to charge (h)/1
  Switch1/1 -> Time to discharge (h)/1
  Gain3/1 -> Switch1/1
  Tapped Delay/1 -> Compare To Zero3/1, Compare To Zero2/1
  Compare To Zero2/1 -> Sum of Elements/1
  Compare To Zero3/1 -> Sum of Elements1/1
  Sum of Elements/1 -> Compare To Constant/1
  Sum of Elements1/1 -> Compare To Constant1/1
  Logical Operator/1 -> Switch/2
  Compare To Zero/1 -> Logical Operator/1
  Compare To Constant/1 -> Logical Operator/2
  Logical Operator1/1 -> Switch1/2
  Compare To Zero1/1 -> Logical Operator1/1
  Compare To Constant1/1 -> Logical Operator1/2
  If1/3 -> Terminator/1

== system BLE_Library/Demodulation, De-whitening, CRC check, PDU/De-whitening, CRC check, Data fields/CRC comparison/CRC comparison ==
  CRC calculated : Inport
  CRC received : Inport  Port=2
  Enable : EnablePort  StatesWhenEnabling=reset
  All bits good : RelationalOperator  Operator===  RndMeth=Nearest  InputSameDT=on
  Constant : Constant  Value=24  SampleTime=Slot_Ts
  Relational Operator : RelationalOperator  Operator===  RndMeth=Nearest  InputSameDT=on
  Total correct bits : Sum  Inputs=1  OutDataTypeStr=double  SaturateOnIntegerOverflow=on  InputSameDT=on
  CRC_OK : Outport  OutputWhenDisabled=reset  InitialOutput=0
  wires:
  CRC received/1 -> Relational Operator/2
  All bits good/1 -> CRC_OK/1
  CRC calculated/1 -> Relational Operator/1
  Total correct bits/1 -> All bits good/1
  Constant/1 -> All bits good/2
  Relational Operator/1 -> Total correct bits/1
